simulink model "Part_2"  (R2017b)
settings: Solver=VariableStepAuto  StartTime=0.0  StopTime=0  RelTol=1e-3
settings Model: Creator=Alireza Rafiee  LastModifiedBy=Alireza Rafiee
settings DataIOCC: ReturnWorkspaceOutputs=on
settings SFSimCC: SimUseLocalCustomCode=on
settings RTWCC: RTWUseLocalCustomCode=on

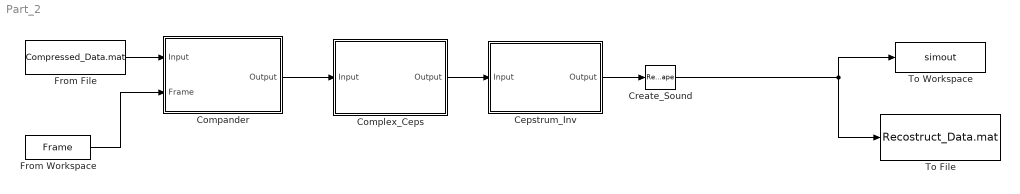
== system Part_2 ==
  Cepstrum_Inv : MATLAB Function  TreatAsAtomicUnit=on
  Compander : MATLAB Function  TreatAsAtomicUnit=on
  Complex_Ceps : MATLAB Function  TreatAsAtomicUnit=on
  Create_Sound : Reshape  OutputDimensions=[400,150]
  From Workspace : FromWorkspace  VariableName=Frame
  From File : FromFile  FileName=Compressed_Data.mat  SampleTime=0
  To File : ToFile  Filename=Recostruct_Data.mat  MatrixName=Compressed_Data  SaveFormat=Timeseries
  To Workspace : ToWorkspace  VariableName=simout  SampleTime=-1
      settings: Save2DSignal=2-D array (concatenate along first dimension)
  wires:
  From File/1 -> Compander/1(Input)
  Compander/1(Output) -> Complex_Ceps/1(Input)
  Complex_Ceps/1(Output) -> Cepstrum_Inv/1(Input)
  Cepstrum_Inv/1(Output) -> Create_Sound/1
  Create_Sound/1 -> To Workspace/1, To File/1
  From Workspace/1 -> Compander/2(Frame)

== matlab function Part_2/Complex_Ceps ==
  data: Input input; Output output
function Output =Complex_Ceps(Input)
    L=0;
    H=0;
    [H,L]=size(Input);
    Output=zeros(H,L);
    Output=2*Input;%Calculate Complex Cepstrum from Real Cepstrum 
    Output(1,:)=Input(1,:);
    Output(H/2,:)=Input(H/2,:);

== matlab function Part_2/Compander ==
  data: Input input; Output output; Frame input
function Output = Compander(Input,Frame)
    L=0;
    H=0;
    [H,L]=size(Input);
    Save_len=H-2;%two end data are pitch_amp and pitch_loc 
    Output=zeros(400,L);
    for i=1:1:L
        for k=1:1:Save_len
            Output(k,i)=Input(k,i); %starting data have neen saved 
        end
        Output(round(Input(Save_len+1,i)),i)=Input(Save_len+2,i);%pitch
    end

== matlab function Part_2/Cepstrum_Inv ==
  data: Input input; Output output
function Output =Cepstrum_Inv(Input)
    L=0;
    H=0;
    [H,L]=size(Input);
    Output=zeros(H,L);
    for i=1:1:L
        Output(:,i)=icceps(Input(:,i),0);%inverse Complex cepstrum
    end
